simulink model "tx2"  (R2022a)
settings: Solver=FixedStepDiscrete  StartTime=0.0  StopTime=3.1e6  FixedStep=1  RelTol=1e-3
undefined symbols (not defined in the file or in its folder): rom_bf1, rom_bf2, rom_bf3, rom_bf4, rom_bf5, rom_bf6, rom_bf7, rom_bf8, rom_pilot_tt
libraries: hdlsllib x809, whdlutilities x460, whdlmod x104, whdledac x26, simulink x3
(part 9 of 27)

== system tx2/Subsystem9/bit_level ==
  note: 此时的输出本身具有一位延迟
  process_data : Inport
  process_valid : Inport  Port=2  OutDataTypeStr=Bus: samplecontrol
  Compare To Constant1 : hdlsllib/Logic and Bit Operations/Compare To Constant  relop=<  const=385  OutDataTypeStr=boolean
      settings: SourceProductBaseCode=SL
  Compare To Constant2 : hdlsllib/Logic and Bit Operations/Compare To Constant  relop===  const=1584+192  OutDataTypeStr=boolean
      settings: SourceProductBaseCode=SL
  Compare To Constant3 : hdlsllib/Logic and Bit Operations/Compare To Constant  relop=>  const=576  OutDataTypeStr=boolean
      settings: SourceProductBaseCode=SL
  Compare To Constant4 : hdlsllib/Logic and Bit Operations/Compare To Constant  relop=<=  const=1584+192  OutDataTypeStr=boolean
      settings: SourceProductBaseCode=SL
  Compare To Constant5 : hdlsllib/Logic and Bit Operations/Compare To Constant  relop=>=  const=792+1  OutDataTypeStr=boolean
      settings: SourceProductBaseCode=SL
  Compare To Constant6 : hdlsllib/Logic and Bit Operations/Compare To Constant  relop=<=  const=1584  OutDataTypeStr=boolean
      settings: SourceProductBaseCode=SL
  Constant : Constant  OutDataTypeStr=boolean
  Constant1 : Constant  Value=72  OutDataTypeStr=uint16
  Constant2 : Constant  Value=0  OutDataTypeStr=boolean
  Constant3 : Constant  Value=0  OutDataTypeStr=fixdt(0,12,0)
  Data Type Conversion1 : DataTypeConversion  OutDataTypeStr=fixdt(0,1,0)  SaturateOnIntegerOverflow=off  RndMeth=Floor
  Data Type Conversion2 : DataTypeConversion  OutDataTypeStr=boolean  SaturateOnIntegerOverflow=off  RndMeth=Floor
  Data Type Conversion3 : DataTypeConversion  OutDataTypeStr=boolean  SaturateOnIntegerOverflow=off  RndMeth=Floor
  Delay1 : Delay  DelayLength=1  InitialCondition=0
  Delay2 : Delay  DelayLength=1  InitialCondition=0
  HDL Counter1 : hdlsllib/Sources/HDL Counter  CountType=Count limited  CountInit=1  CountStep=1  CountMax=1584  CountFromType=Initial value  CountFrom=1  CountResetPort=on  CountLoadPort=off  CountEnbPort=on  CountDirPort=off  CountHitOutputPort=off  CountDataType=Unsigned  CountWordLen=12  CountFracLen=0  CountSampTime=1
  HDL Counter2 : hdlsllib/Sources/HDL Counter  CountType=Count limited  CountInit=1  CountStep=1  CountMax=792  CountFromType=Initial value  CountFrom=1  CountResetPort=on  CountLoadPort=off  CountEnbPort=on  CountDirPort=off  CountHitOutputPort=off  CountDataType=Unsigned  CountWordLen=12  CountFracLen=0  CountSampTime=1
  HDL Counter4 : hdlsllib/Sources/HDL Counter  CountType=Count limited  CountInit=1  CountStep=1  CountMax=4096-1  CountFromType=Initial value  CountFrom=1  CountResetPort=on  CountLoadPort=off  CountEnbPort=on  CountDirPort=off  CountHitOutputPort=off  CountDataType=Unsigned  CountWordLen=12  CountFracLen=0  CountSampTime=1
  HDL Counter5 : hdlsllib/Sources/HDL Counter  CountType=Count limited  CountInit=0  CountStep=1  CountMax=1  CountFromType=Initial value  CountFrom=0  CountResetPort=on  CountLoadPort=off  CountEnbPort=on  CountDirPort=off  CountHitOutputPort=off  CountDataType=Unsigned  CountWordLen=1  CountFracLen=0  CountSampTime=1
  Logical Operator : Logic  Operator=OR  AllPortsSameDT=off  OutDataTypeStr=boolean
  Logical Operator{1,3,7..8} (4 alike) : Logic  Operator=NOT  AllPortsSameDT=off  OutDataTypeStr=boolean
  Logical Operator{2,4..6} (4 alike) : Logic  AllPortsSameDT=off  OutDataTypeStr=boolean
  Mux : Mux  Inputs=2
  NR CRC Encoder : whdledac/NR CRC Encoder  CRCType=CRC16  EnableCRCMaskPort=off  SimulateUsing=Code generation
      settings: SourceProductBaseCode=LH
  NR LDPC Encoder2 : whdledac/NR LDPC Encoder
      settings: SourceProductBaseCode=LH
  Sample Control Bus Creator : whdlutilities/Sample Control Bus Creator
      settings: SourceProductBaseCode=LH
  Sample Control Bus Selector : whdlutilities/Sample Control Bus Selector  OutputSignals=start,end,valid
      settings: SourceProductBaseCode=LH
  Sample Control Bus Selector1 : whdlutilities/Sample Control Bus Selector  OutputSignals=start,end,valid
      settings: SourceProductBaseCode=LH
  Simple Dual Port RAM1 : hdlsllib/HDL RAMs/Simple Dual Port RAM  ram_size=12
      settings: SourceProductBaseCode=SL
  Subsystem : Subsystem
  Switch : Switch  Criteria=u2 ~= 0  SaturateOnIntegerOverflow=off  InputSameDT=off
  Switch1 : Switch  Criteria=u2 ~= 0  SaturateOnIntegerOverflow=off  InputSameDT=off
  Switch2 : Switch  Criteria=u2 ~= 0  SaturateOnIntegerOverflow=off  InputSameDT=off
  ctrl_gen : Subsystem
  valid_recover : Subsystem
  bit_level_process : Outport  OutDataTypeStr=boolean
  "bit_level_ctrl_process " : Outport  Port=2  OutDataTypeStr=Bus: samplecontrol
  wires:
  ctrl_gen/1(data_out) -> bit_level_process/1  "INTERLEAVE"
  process_valid/1 -> NR CRC Encoder/2
  Delay2/1 -> ctrl_gen/2(select_valid)
  Delay1/1 -> Mux/2
  Compare To Constant4/1 -> Logical Operator2/2
  Mux/1 -> ctrl_gen/1(data_in)
  Sample Control Bus Creator/1 -> NR LDPC Encoder2/2
  NR CRC Encoder/2 -> Sample Control Bus Selector/1
  Compare To Constant1/1 -> Logical Operator/1
  Compare To Constant2/1 -> HDL Counter5/2
  Constant2/1 -> Switch/3
  Compare To Constant6/1 -> Logical Operator6/2
  HDL Counter4/1 -> Compare To Constant2/1, Compare To Constant3/1, Compare To Constant4/1, Compare To Constant1/1  "wr_addr"
  Data Type Conversion1/1 -> Simple Dual Port RAM1/1  "wr_din"
  Compare To Constant5/1 -> Logical Operator6/1
  Logical Operator5/1 -> Simple Dual Port RAM1/3, Switch1/2, HDL Counter1/2  "wr_en"
  Compare To Constant3/1 -> Logical Operator/2
  Subsystem/1(end_out) -> valid_recover/3(end_in)
  process_data/1 -> NR CRC Encoder/1
  Data Type Conversion2/1 -> HDL Counter4/1
  Switch1/1 -> Simple Dual Port RAM1/2  "wr_addr"
  Logical Operator6/1 -> Switch/2, Delay2/1, Logical Operator7/1, Switch2/2, HDL Counter2/2
  Logical Operator1/1 -> HDL Counter1/1
  valid_recover/1(data_out) -> NR LDPC Encoder2/1
  NR LDPC Encoder2/2 -> Sample Control Bus Selector1/1
  HDL Counter1/1 -> Compare To Constant5/1, Compare To Constant6/1, Switch1/1
  Switch2/1 -> Simple Dual Port RAM1/4  "rd_addr"
  valid_recover/4(valid_out) -> Sample Control Bus Creator/3
  Logical Operator/1 -> Logical Operator2/1
  Logical Operator4/1 -> Logical Operator5/2
  Logical Operator3/1 -> Logical Operator4/1
  Logical Operator7/1 -> HDL Counter2/1
  Logical Operator2/1 -> Logical Operator5/1
  Sample Control Bus Selector1/3 -> Logical Operator4/2, Logical Operator1/1, Logical Operator8/1, HDL Counter4/2  "<valid>"
  valid_recover/3(end_out) -> Sample Control Bus Creator/2
  valid_recover/2(start_out) -> Sample Control Bus Creator/1
  Sample Control Bus Selector/1 -> valid_recover/2(start_in)  "<start>"
  Simple Dual Port RAM1/1 -> Data Type Conversion3/1
  NR LDPC Encoder2/1 -> Data Type Conversion1/1, Switch/1  "LDPC"
  Sample Control Bus Selector/2 -> Subsystem/1(end_in)  "<end>"
  Logical Operator8/1 -> HDL Counter5/1
  HDL Counter2/1 -> Switch2/1  "rd_addr"
  Constant1/1 -> NR LDPC Encoder2/4
  ctrl_gen/2(ctrl_out) -> "bit_level_ctrl_process "/1
  NR CRC Encoder/1 -> valid_recover/1(data_in)  "CRC"
  Constant3/1 -> Switch1/3, Switch2/3
  Constant/1 -> NR LDPC Encoder2/3
  Data Type Conversion3/1 -> Mux/1
  HDL Counter5/1 -> Data Type Conversion2/1, Logical Operator3/1  "loop_ctrl"
  Switch/1 -> Delay1/1

== system tx2/Subsystem9/mapping_process_L1 ==
  data_in : Inport  OutDataTypeStr=boolean
  mapping_ctrl : Inport  Port=2  OutDataTypeStr=Bus: samplecontrol
  Constant : Constant  Value=sqrt(2)/2  OutDataTypeStr=fixdt(1,16,14)
  Constant1 : Constant  Value=-sqrt(2)/2  OutDataTypeStr=fixdt(1,16,14)
  Constant2 : Constant  Value=0  OutDataTypeStr=uint8
  Constant3 : Constant  Value=0  OutDataTypeStr=fixdt(1,16,14)
  Delay : Delay  DelayLength=1  InitialCondition=0  ShowEnablePort=on
      settings: InputPortMap=u0,e6
  Delay{1,5..8,10..12} (8 alike) : Delay  DelayLength=1  InitialCondition=0
  Delay{3..4,9,13} (4 alike) : Delay  InitialCondition=0
  Delay2 : Delay  DelayLength=1  InitialCondition=0  ShowEnablePort=on
      settings: InputPortMap=u0,e6
  Demux : Demux  Outputs=2
  Logical Operator : Logic  Operator=OR  AllPortsSameDT=off  OutDataTypeStr=boolean
  Logical Operator1 : Logic  AllPortsSameDT=off  OutDataTypeStr=boolean
  Logical Operator13 : Logic  Operator=NOT  AllPortsSameDT=off  OutDataTypeStr=boolean
  Real-Imag to Complex : RealImagToComplex
  Real-Imag to Complex1 : RealImagToComplex
  Sample Control Bus Creator : whdlutilities/Sample Control Bus Creator
      settings: SourceProductBaseCode=LH
  Sample Control Bus Creator1 : whdlutilities/Sample Control Bus Creator
      settings: SourceProductBaseCode=LH
  Sample Control Bus Selector : whdlutilities/Sample Control Bus Selector  OutputSignals=start,end,valid
      settings: SourceProductBaseCode=LH
  Switch{,1..3} (4 alike) : Switch  Criteria=u2 ~= 0  SaturateOnIntegerOverflow=off  InputSameDT=off
  "divide6 " : hdlsllib/Sources/HDL Counter  CountType=Count limited  CountInit=1  CountStep=1  CountMax=12  CountFromType=Initial value  CountFrom=1  CountResetPort=on  CountLoadPort=off  CountEnbPort=on  CountDirPort=off  CountHitOutputPort=on  CountDataType=Unsigned  CountWordLen=8  CountFracLen=0  CountSampTime=1
  divide6 1 : hdlsllib/Sources/HDL Counter  CountType=Count limited  CountInit=1  CountStep=1  CountMax=6*12  CountFromType=Initial value  CountFrom=1  CountResetPort=on  CountLoadPort=off  CountEnbPort=on  CountDirPort=off  CountHitOutputPort=off  CountDataType=Unsigned  CountWordLen=8  CountFracLen=0  CountSampTime=1
  data_out : Outport  VectorParamsAs1DForOutWhenUnconnected=off
      settings: SignalType=complex
  ctrl_mapping : Outport  Port=2  OutDataTypeStr=Bus: samplecontrol  VectorParamsAs1DForOutWhenUnconnected=off
  RB_ctrl : Outport  Port=3  OutDataTypeStr=Bus: samplecontrol  VectorParamsAs1DForOutWhenUnconnected=off
  RB_id : Outport  Port=4  OutDataTypeStr=uint8  VectorParamsAs1DForOutWhenUnconnected=off
  wires:
  Constant1/1 -> Switch1/1, Switch/1
  Constant/1 -> Switch/3, Switch1/3
  Delay13/1 -> Switch3/2
  Real-Imag to Complex1/1 -> Switch3/3
  Constant3/1 -> Real-Imag to Complex1/1, Real-Imag to Complex1/2
  Switch3/1 -> data_out/1
  data_in/1 -> Delay/1  "data_with_CP"
  Sample Control Bus Creator1/1 -> RB_ctrl/1
  Delay7/1 -> RB_id/1
  Delay5/1 -> ctrl_mapping/1
  Delay12/1 -> Sample Control Bus Creator1/3
  Delay11/1 -> Sample Control Bus Creator1/2
  Delay8/1 -> Sample Control Bus Creator1/1
  Logical Operator1/1 -> Delay8/1
  Delay10/1 -> Logical Operator/1
  Delay9/1 -> Logical Operator/2
  Logical Operator/1 -> Logical Operator1/2
  Delay6/1 -> Switch3/1
  Constant2/1 -> Switch2/3
  Switch2/1 -> Delay7/1
  Delay4/1 -> Logical Operator1/1, Switch2/2, Delay12/1, "divide6 "/2, Logical Operator13/1
  divide6 1/1 -> Switch2/1  "RB_id"
  Sample Control Bus Creator/1 -> Delay3/1
  Sample Control Bus Selector/3 -> Delay/2, Delay1/1, Delay4/1, Sample Control Bus Creator/3  "<valid>"
  Sample Control Bus Selector/2 -> Sample Control Bus Creator/2  "<end>"
  Sample Control Bus Selector/1 -> Sample Control Bus Creator/1, Delay9/1  "<start>"
  Logical Operator13/1 -> "divide6 "/1, divide6 1/1
  "divide6 "/2 -> Delay10/1, Delay11/1, divide6 1/2  "count6"
  mapping_ctrl/1 -> Sample Control Bus Selector/1
  Delay1/1 -> Delay13/1, Delay2/2
  Delay3/1 -> Delay5/1
  Delay2/1 -> Delay6/1
  Real-Imag to Complex/1 -> Delay2/1
  Demux/2 -> Switch1/2
  Demux/1 -> Switch/2
  Delay/1 -> Demux/1
  Switch/1 -> Real-Imag to Complex/1
  Switch1/1 -> Real-Imag to Complex/2

== system tx2/transport_block1/Subsystem10 ==
  data_in : Inport
  select_valid : Inport  Port=2  OutDataTypeStr=boolean
  Constant : Constant  Value=0  OutDataTypeStr=boolean
  Switch : Switch  Criteria=u2 ~= 0  SaturateOnIntegerOverflow=off  InputSameDT=off
  ctrl_gen : Subsystem
  data_out : Outport
  ctrl_out : Outport  Port=2
  wires:
  Switch/1 -> ctrl_gen/1(data_in)
  Constant/1 -> Switch/3
  select_valid/1 -> ctrl_gen/2(valid_in), Switch/2
  ctrl_gen/1(data_out) -> data_out/1
  ctrl_gen/2(ctrl_out) -> ctrl_out/1
  data_in/1 -> Switch/1

== system tx2/transport_block1/Subsystem11 ==
  data_in : Inport
  select_valid : Inport  Port=2  OutDataTypeStr=boolean
  Constant : Constant  Value=0  OutDataTypeStr=boolean
  Switch : Switch  Criteria=u2 ~= 0  SaturateOnIntegerOverflow=off  InputSameDT=off
  ctrl_gen : Subsystem
  data_out : Outport
  ctrl_out : Outport  Port=2
  wires:
  data_in/1 -> Switch/1
  ctrl_gen/2(ctrl_out) -> ctrl_out/1
  ctrl_gen/1(data_out) -> data_out/1
  select_valid/1 -> Switch/2, ctrl_gen/2(valid_in)
  Constant/1 -> Switch/3
  Switch/1 -> ctrl_gen/1(data_in)

== system tx2/transport_block1/Subsystem12 ==
  data_in : Inport
  select_valid : Inport  Port=2  OutDataTypeStr=boolean
  Constant : Constant  Value=0  OutDataTypeStr=boolean
  Switch : Switch  Criteria=u2 ~= 0  SaturateOnIntegerOverflow=off  InputSameDT=off
  ctrl_gen : Subsystem
  data_out : Outport
  ctrl_out : Outport  Port=2
  wires:
  Switch/1 -> ctrl_gen/1(data_in)
  Constant/1 -> Switch/3
  select_valid/1 -> ctrl_gen/2(valid_in), Switch/2
  ctrl_gen/1(data_out) -> data_out/1
  ctrl_gen/2(ctrl_out) -> ctrl_out/1
  data_in/1 -> Switch/1

== system tx2/transport_block1/Subsystem13 ==
  data_in : Inport
  select_valid : Inport  Port=2  OutDataTypeStr=boolean
  Constant : Constant  Value=0  OutDataTypeStr=boolean
  Switch : Switch  Criteria=u2 ~= 0  SaturateOnIntegerOverflow=off  InputSameDT=off
  ctrl_gen : Subsystem
  data_out : Outport
  ctrl_out : Outport  Port=2
  wires:
  data_in/1 -> Switch/1
  ctrl_gen/2(ctrl_out) -> ctrl_out/1
  ctrl_gen/1(data_out) -> data_out/1
  select_valid/1 -> Switch/2, ctrl_gen/2(valid_in)
  Constant/1 -> Switch/3
  Switch/1 -> ctrl_gen/1(data_in)

== system tx2/transport_block1/Subsystem14 ==
  data_in : Inport
  select_valid : Inport  Port=2  OutDataTypeStr=boolean
  Constant : Constant  Value=0  OutDataTypeStr=boolean
  Switch : Switch  Criteria=u2 ~= 0  SaturateOnIntegerOverflow=off  InputSameDT=off
  ctrl_gen : Subsystem
  data_out : Outport
  ctrl_out : Outport  Port=2
  wires:
  Switch/1 -> ctrl_gen/1(data_in)
  Constant/1 -> Switch/3
  select_valid/1 -> ctrl_gen/2(valid_in), Switch/2
  ctrl_gen/1(data_out) -> data_out/1
  ctrl_gen/2(ctrl_out) -> ctrl_out/1
  data_in/1 -> Switch/1

== system tx2/transport_block1/Subsystem2 ==
  data_in : Inport
  select_valid : Inport  Port=2  OutDataTypeStr=boolean
  Constant : Constant  Value=0  OutDataTypeStr=boolean
  Switch : Switch  Criteria=u2 ~= 0  SaturateOnIntegerOverflow=off  InputSameDT=off
  ctrl_gen : Subsystem
  data_out : Outport
  ctrl_out : Outport  Port=2
  wires:
  data_in/1 -> Switch/1
  ctrl_gen/2(ctrl_out) -> ctrl_out/1
  ctrl_gen/1(data_out) -> data_out/1
  select_valid/1 -> Switch/2, ctrl_gen/2(valid_in)
  Constant/1 -> Switch/3
  Switch/1 -> ctrl_gen/1(data_in)

== system tx2/transport_block1/Subsystem3 ==
  data_in : Inport
  select_valid : Inport  Port=2  OutDataTypeStr=boolean
  Constant : Constant  Value=0  OutDataTypeStr=boolean
  Switch : Switch  Criteria=u2 ~= 0  SaturateOnIntegerOverflow=off  InputSameDT=off
  ctrl_gen : Subsystem
  data_out : Outport
  ctrl_out : Outport  Port=2
  wires:
  Switch/1 -> ctrl_gen/1(data_in)
  Constant/1 -> Switch/3
  select_valid/1 -> ctrl_gen/2(valid_in), Switch/2
  ctrl_gen/1(data_out) -> data_out/1
  ctrl_gen/2(ctrl_out) -> ctrl_out/1
  data_in/1 -> Switch/1

== system tx2/transport_block1/Subsystem4 ==
  data_in : Inport
  select_valid : Inport  Port=2  OutDataTypeStr=boolean
  Constant : Constant  Value=0  OutDataTypeStr=boolean
  Switch : Switch  Criteria=u2 ~= 0  SaturateOnIntegerOverflow=off  InputSameDT=off
  ctrl_gen : Subsystem
  data_out : Outport
  ctrl_out : Outport  Port=2
  wires:
  data_in/1 -> Switch/1
  ctrl_gen/2(ctrl_out) -> ctrl_out/1
  ctrl_gen/1(data_out) -> data_out/1
  select_valid/1 -> Switch/2, ctrl_gen/2(valid_in)
  Constant/1 -> Switch/3
  Switch/1 -> ctrl_gen/1(data_in)

== system tx2/transport_block1/Subsystem5 ==
  data_in : Inport
  select_valid : Inport  Port=2  OutDataTypeStr=boolean
  Constant : Constant  Value=0  OutDataTypeStr=boolean
  Switch : Switch  Criteria=u2 ~= 0  SaturateOnIntegerOverflow=off  InputSameDT=off
  ctrl_gen : Subsystem
  data_out : Outport
  ctrl_out : Outport  Port=2
  wires:
  Switch/1 -> ctrl_gen/1(data_in)
  Constant/1 -> Switch/3
  select_valid/1 -> ctrl_gen/2(valid_in), Switch/2
  ctrl_gen/1(data_out) -> data_out/1
  ctrl_gen/2(ctrl_out) -> ctrl_out/1
  data_in/1 -> Switch/1

== system tx2/transport_block1/Subsystem6 ==
  data_in : Inport
  select_valid : Inport  Port=2  OutDataTypeStr=boolean
  Constant : Constant  Value=0  OutDataTypeStr=boolean
  Switch : Switch  Criteria=u2 ~= 0  SaturateOnIntegerOverflow=off  InputSameDT=off
  ctrl_gen : Subsystem
  data_out : Outport
  ctrl_out : Outport  Port=2
  wires:
  data_in/1 -> Switch/1
  ctrl_gen/2(ctrl_out) -> ctrl_out/1
  ctrl_gen/1(data_out) -> data_out/1
  select_valid/1 -> Switch/2, ctrl_gen/2(valid_in)
  Constant/1 -> Switch/3
  Switch/1 -> ctrl_gen/1(data_in)

== system tx2/transport_block1/Subsystem7 ==
  data_in : Inport
  select_valid : Inport  Port=2  OutDataTypeStr=boolean
  Constant : Constant  Value=0  OutDataTypeStr=boolean
  Switch : Switch  Criteria=u2 ~= 0  SaturateOnIntegerOverflow=off  InputSameDT=off
  ctrl_gen : Subsystem
  data_out : Outport
  ctrl_out : Outport  Port=2
  wires:
  Switch/1 -> ctrl_gen/1(data_in)
  Constant/1 -> Switch/3
  select_valid/1 -> ctrl_gen/2(valid_in), Switch/2
  ctrl_gen/1(data_out) -> data_out/1
  ctrl_gen/2(ctrl_out) -> ctrl_out/1
  data_in/1 -> Switch/1

== system tx2/transport_block1/Subsystem8 ==
  data_in : Inport
  select_valid : Inport  Port=2  OutDataTypeStr=boolean
  Constant : Constant  Value=0  OutDataTypeStr=boolean
  Switch : Switch  Criteria=u2 ~= 0  SaturateOnIntegerOverflow=off  InputSameDT=off
  ctrl_gen : Subsystem
  data_out : Outport
  ctrl_out : Outport  Port=2
  wires:
  data_in/1 -> Switch/1
  ctrl_gen/2(ctrl_out) -> ctrl_out/1
  ctrl_gen/1(data_out) -> data_out/1
  select_valid/1 -> Switch/2, ctrl_gen/2(valid_in)
  Constant/1 -> Switch/3
  Switch/1 -> ctrl_gen/1(data_in)

== system tx2/transport_block1/Subsystem9 ==
  data_in : Inport
  select_valid : Inport  Port=2  OutDataTypeStr=boolean
  Constant : Constant  Value=0  OutDataTypeStr=boolean
  Switch : Switch  Criteria=u2 ~= 0  SaturateOnIntegerOverflow=off  InputSameDT=off
  ctrl_gen : Subsystem
  data_out : Outport
  ctrl_out : Outport  Port=2
  wires:
  data_in/1 -> Switch/1
  ctrl_gen/2(ctrl_out) -> ctrl_out/1
  ctrl_gen/1(data_out) -> data_out/1
  select_valid/1 -> Switch/2, ctrl_gen/2(valid_in)
  Constant/1 -> Switch/3
  Switch/1 -> ctrl_gen/1(data_in)

== system tx2/transport_block1/process_selector ==
  enb : Inport
  rst : Inport  Port=2  OutDataTypeStr=boolean
  Constant : Constant  Value=0  OutDataTypeStr=uint8
  HDL Counter : hdlsllib/Sources/HDL Counter  CountType=Count limited  CountInit=1  CountStep=1  CountMax=transblock_len  CountFromType=Initial value  CountFrom=1  CountResetPort=on  CountLoadPort=off  CountEnbPort=on  CountDirPort=off  CountHitOutputPort=on  CountDataType=Unsigned  CountWordLen=10  CountFracLen=0  CountSampTime=1
  HDL Counter1 : hdlsllib/Sources/HDL Counter  CountType=Count limited  CountInit=1  CountStep=1  CountMax=process_len  CountFromType=Initial value  CountFrom=1  CountResetPort=on  CountLoadPort=off  CountEnbPort=on  CountDirPort=off  CountHitOutputPort=off  CountDataType=Unsigned  CountWordLen=8  CountFracLen=0  CountSampTime=1
  Switch : Switch  Criteria=u2 ~= 0  SaturateOnIntegerOverflow=off  InputSameDT=off
  selector : Outport
  wires:
  rst/1 -> HDL Counter1/1, HDL Counter/1
  HDL Counter1/1 -> Switch/1
  enb/1 -> HDL Counter/2, Switch/2
  HDL Counter/1 -> ?
  Switch/1 -> selector/1
  Constant/1 -> Switch/3
  HDL Counter/2 -> HDL Counter1/2

== system tx2/Subsystem1/BF/rom_bf1 ==
  address : Inport
  read_en : Inport  Port=2
  HDL ROM : Subsystem
  InputReg : Delay  DelayLength=1  ShowEnablePort=on
      settings: InputPortMap=u0,e6
  data_out : Outport
  wires:
  address/1 -> InputReg/1
  InputReg/1 -> HDL ROM/1(rom_address)
  read_en/1 -> InputReg/2
  HDL ROM/1(data_out) -> data_out/1

== system tx2/Subsystem1/BF/rom_bf2 ==
  address : Inport
  read_en : Inport  Port=2
  HDL ROM : Subsystem
  InputReg : Delay  DelayLength=1  ShowEnablePort=on
      settings: InputPortMap=u0,e6
  data_out : Outport
  wires:
  HDL ROM/1(data_out) -> data_out/1
  read_en/1 -> InputReg/2
  InputReg/1 -> HDL ROM/1(rom_address)
  address/1 -> InputReg/1

== system tx2/Subsystem1/BF/rom_bf3 ==
  address : Inport
  read_en : Inport  Port=2
  HDL ROM : Subsystem
  InputReg : Delay  DelayLength=1  ShowEnablePort=on
      settings: InputPortMap=u0,e6
  data_out : Outport
  wires:
  address/1 -> InputReg/1
  InputReg/1 -> HDL ROM/1(rom_address)
  read_en/1 -> InputReg/2
  HDL ROM/1(data_out) -> data_out/1

== system tx2/Subsystem1/BF/rom_bf4 ==
  address : Inport
  read_en : Inport  Port=2
  HDL ROM : Subsystem
  InputReg : Delay  DelayLength=1  ShowEnablePort=on
      settings: InputPortMap=u0,e6
  data_out : Outport
  wires:
  HDL ROM/1(data_out) -> data_out/1
  read_en/1 -> InputReg/2
  InputReg/1 -> HDL ROM/1(rom_address)
  address/1 -> InputReg/1

== system tx2/Subsystem1/BF/rom_bf5 ==
  address : Inport
  read_en : Inport  Port=2
  HDL ROM : Subsystem
  InputReg : Delay  DelayLength=1  ShowEnablePort=on
      settings: InputPortMap=u0,e6
  data_out : Outport
  wires:
  address/1 -> InputReg/1
  InputReg/1 -> HDL ROM/1(rom_address)
  read_en/1 -> InputReg/2
  HDL ROM/1(data_out) -> data_out/1

== system tx2/Subsystem1/BF/rom_bf6 ==
  address : Inport
  read_en : Inport  Port=2
  HDL ROM : Subsystem
  InputReg : Delay  DelayLength=1  ShowEnablePort=on
      settings: InputPortMap=u0,e6
  data_out : Outport
  wires:
  HDL ROM/1(data_out) -> data_out/1
  read_en/1 -> InputReg/2
  InputReg/1 -> HDL ROM/1(rom_address)
  address/1 -> InputReg/1

== system tx2/Subsystem1/BF/rom_bf7 ==
  address : Inport
  read_en : Inport  Port=2
  HDL ROM : Subsystem
  InputReg : Delay  DelayLength=1  ShowEnablePort=on
      settings: InputPortMap=u0,e6
  data_out : Outport
  wires:
  address/1 -> InputReg/1
  InputReg/1 -> HDL ROM/1(rom_address)
  read_en/1 -> InputReg/2
  HDL ROM/1(data_out) -> data_out/1

== system tx2/Subsystem1/BF/rom_bf8 ==
  address : Inport
  read_en : Inport  Port=2
  HDL ROM : Subsystem
  InputReg : Delay  DelayLength=1  ShowEnablePort=on
      settings: InputPortMap=u0,e6
  data_out : Outport
  wires:
  HDL ROM/1(data_out) -> data_out/1
  read_en/1 -> InputReg/2
  InputReg/1 -> HDL ROM/1(rom_address)
  address/1 -> InputReg/1

== system tx2/Subsystem1/OFDM_process1/OFDM_process1_bf1 ==
  data : Inport
  BF_ctrl : Inport  Port=2
  OFDM_BF1 : Subsystem
  ctrl_gen : Subsystem
  OFDM_process : Outport
  OFDM_ctrl_process : Outport  Port=2
  wires:
  OFDM_BF1/1(data_out) -> ctrl_gen/1(data_in)
  OFDM_BF1/2(valid_out) -> ctrl_gen/2(valid_in)
  data/1 -> OFDM_BF1/1(data)
  ctrl_gen/2(ctrl_out) -> OFDM_ctrl_process/1  "OFDM_ctrl_bf1_process1"
  BF_ctrl/1 -> OFDM_BF1/2(OFDM_ctrl)
  ctrl_gen/1(data_out) -> OFDM_process/1  "OFDM_bf1_process1"

== system tx2/Subsystem1/OFDM_process1/OFDM_process1_bf2 ==
  data : Inport
  BF_ctrl : Inport  Port=2
  OFDM_BF1 : Subsystem
  ctrl_gen : Subsystem
  OFDM_process : Outport
  OFDM_ctrl_process : Outport  Port=2
  wires:
  ctrl_gen/1(data_out) -> OFDM_process/1  "OFDM_bf1_process1"
  BF_ctrl/1 -> OFDM_BF1/2(OFDM_ctrl)
  ctrl_gen/2(ctrl_out) -> OFDM_ctrl_process/1  "OFDM_ctrl_bf1_process1"
  data/1 -> OFDM_BF1/1(data)
  OFDM_BF1/2(valid_out) -> ctrl_gen/2(valid_in)
  OFDM_BF1/1(data_out) -> ctrl_gen/1(data_in)

== system tx2/Subsystem1/OFDM_process1/OFDM_process1_bf3 ==
  data : Inport
  BF_ctrl : Inport  Port=2
  OFDM_BF1 : Subsystem
  ctrl_gen : Subsystem
  OFDM_process : Outport
  OFDM_ctrl_process : Outport  Port=2
  wires:
  OFDM_BF1/1(data_out) -> ctrl_gen/1(data_in)
  OFDM_BF1/2(valid_out) -> ctrl_gen/2(valid_in)
  data/1 -> OFDM_BF1/1(data)
  ctrl_gen/2(ctrl_out) -> OFDM_ctrl_process/1  "OFDM_ctrl_bf1_process1"
  BF_ctrl/1 -> OFDM_BF1/2(OFDM_ctrl)
  ctrl_gen/1(data_out) -> OFDM_process/1  "OFDM_bf1_process1"

== system tx2/Subsystem1/OFDM_process1/OFDM_process1_bf4 ==
  data : Inport
  BF_ctrl : Inport  Port=2
  OFDM_BF1 : Subsystem
  ctrl_gen : Subsystem
  OFDM_process : Outport
  OFDM_ctrl_process : Outport  Port=2
  wires:
  ctrl_gen/1(data_out) -> OFDM_process/1  "OFDM_bf1_process1"
  BF_ctrl/1 -> OFDM_BF1/2(OFDM_ctrl)
  ctrl_gen/2(ctrl_out) -> OFDM_ctrl_process/1  "OFDM_ctrl_bf1_process1"
  data/1 -> OFDM_BF1/1(data)
  OFDM_BF1/2(valid_out) -> ctrl_gen/2(valid_in)
  OFDM_BF1/1(data_out) -> ctrl_gen/1(data_in)

== system tx2/Subsystem1/OFDM_process1/OFDM_process1_bf5 ==
  data : Inport
  BF_ctrl : Inport  Port=2
  OFDM_BF1 : Subsystem
  ctrl_gen : Subsystem
  OFDM_process : Outport
  OFDM_ctrl_process : Outport  Port=2
  wires:
  OFDM_BF1/1(data_out) -> ctrl_gen/1(data_in)
  OFDM_BF1/2(valid_out) -> ctrl_gen/2(valid_in)
  data/1 -> OFDM_BF1/1(data)
  ctrl_gen/2(ctrl_out) -> OFDM_ctrl_process/1  "OFDM_ctrl_bf1_process1"
  BF_ctrl/1 -> OFDM_BF1/2(OFDM_ctrl)
  ctrl_gen/1(data_out) -> OFDM_process/1  "OFDM_bf1_process1"

== system tx2/Subsystem1/OFDM_process1/OFDM_process1_bf6 ==
  data : Inport
  BF_ctrl : Inport  Port=2
  OFDM_BF1 : Subsystem
  ctrl_gen : Subsystem
  OFDM_process : Outport
  OFDM_ctrl_process : Outport  Port=2
  wires:
  ctrl_gen/1(data_out) -> OFDM_process/1  "OFDM_bf1_process1"
  BF_ctrl/1 -> OFDM_BF1/2(OFDM_ctrl)
  ctrl_gen/2(ctrl_out) -> OFDM_ctrl_process/1  "OFDM_ctrl_bf1_process1"
  data/1 -> OFDM_BF1/1(data)
  OFDM_BF1/2(valid_out) -> ctrl_gen/2(valid_in)
  OFDM_BF1/1(data_out) -> ctrl_gen/1(data_in)

== system tx2/Subsystem1/OFDM_process1/OFDM_process1_bf7 ==
  data : Inport
  BF_ctrl : Inport  Port=2
  OFDM_BF1 : Subsystem
  ctrl_gen : Subsystem
  OFDM_process : Outport
  OFDM_ctrl_process : Outport  Port=2
  wires:
  OFDM_BF1/1(data_out) -> ctrl_gen/1(data_in)
  OFDM_BF1/2(valid_out) -> ctrl_gen/2(valid_in)
  data/1 -> OFDM_BF1/1(data)
  ctrl_gen/2(ctrl_out) -> OFDM_ctrl_process/1  "OFDM_ctrl_bf1_process1"
  BF_ctrl/1 -> OFDM_BF1/2(OFDM_ctrl)
  ctrl_gen/1(data_out) -> OFDM_process/1  "OFDM_bf1_process1"

== system tx2/Subsystem1/OFDM_process1/OFDM_process1_bf8 ==
  data : Inport
  BF_ctrl : Inport  Port=2
  OFDM_BF1 : Subsystem
  ctrl_gen : Subsystem
  OFDM_process : Outport
  OFDM_ctrl_process : Outport  Port=2
  wires:
  ctrl_gen/1(data_out) -> OFDM_process/1  "OFDM_bf1_process1"
  BF_ctrl/1 -> OFDM_BF1/2(OFDM_ctrl)
  ctrl_gen/2(ctrl_out) -> OFDM_ctrl_process/1  "OFDM_ctrl_bf1_process1"
  data/1 -> OFDM_BF1/1(data)
  OFDM_BF1/2(valid_out) -> ctrl_gen/2(valid_in)
  OFDM_BF1/1(data_out) -> ctrl_gen/1(data_in)

== system tx2/Subsystem1/bit_level/Subsystem ==
  end_in : Inport  OutDataTypeStr=boolean
  Data Type Conversion : DataTypeConversion  OutDataTypeStr=boolean  SaturateOnIntegerOverflow=off  RndMeth=Floor
  HDL Counter : hdlsllib/Sources/HDL Counter  CountType=Count limited  CountInit=1  CountStep=1  CountMax=192  CountFromType=Initial value  CountFrom=1  CountResetPort=on  CountLoadPort=off  CountEnbPort=off  CountDirPort=off  CountHitOutputPort=on  CountDataType=Unsigned  CountWordLen=8  CountFracLen=0  CountSampTime=1
  HDL Counter1 : hdlsllib/Sources/HDL Counter  CountType=Count limited  CountInit=0  CountStep=1  CountMax=1  CountFromType=Initial value  CountFrom=0  CountResetPort=on  CountLoadPort=off  CountEnbPort=on  CountDirPort=off  CountHitOutputPort=off  CountDataType=Unsigned  CountWordLen=1  CountFracLen=0  CountSampTime=1
  Logical Operator : Logic  AllPortsSameDT=off  OutDataTypeStr=boolean
  end_out : Outport  OutDataTypeStr=boolean
  wires:
  HDL Counter1/1 -> Data Type Conversion/1
  end_in/1 -> HDL Counter/1, HDL Counter1/2
  Data Type Conversion/1 -> Logical Operator/2
  HDL Counter/2 -> Logical Operator/1, HDL Counter1/1
  Logical Operator/1 -> end_out/1

== system tx2/Subsystem1/bit_level/ctrl_gen ==
  data_in : Inport
  select_valid : Inport  Port=2  OutDataTypeStr=boolean
  Constant : Constant  Value=0  OutDataTypeStr=boolean
  Switch : Switch  Criteria=u2 ~= 0  SaturateOnIntegerOverflow=off  InputSameDT=off
  ctrl_gen : Subsystem
  data_out : Outport
  ctrl_out : Outport  Port=2
  wires:
  Switch/1 -> ctrl_gen/1(data_in)
  Constant/1 -> Switch/3
  select_valid/1 -> ctrl_gen/2(valid_in), Switch/2
  ctrl_gen/1(data_out) -> data_out/1
  ctrl_gen/2(ctrl_out) -> ctrl_out/1
  data_in/1 -> Switch/1

== system tx2/Subsystem1/bit_level/valid_recover ==
  data_in : Inport
  start_in : Inport  Port=2
  end_in : Inport  Port=3
  Constant : Constant  OutDataTypeStr=boolean
  Constant1 : Constant  Value=0  OutDataTypeStr=boolean
  Constant2 : Constant  OutDataTypeStr=boolean
  Constant3 : Constant  Value=0  OutDataTypeStr=boolean
  Constant4 : Constant  OutDataTypeStr=boolean
  Constant5 : Constant  Value=0  OutDataTypeStr=boolean
  Delay{,1..4} (5 alike) : Delay  DelayLength=1  InitialCondition=0
  Logical Operator1 : Logic  Operator=OR  AllPortsSameDT=off  OutDataTypeStr=boolean
  Logical Operator2 : Logic  AllPortsSameDT=off  OutDataTypeStr=boolean
  Switch : Switch  Criteria=u2 ~= 0  SaturateOnIntegerOverflow=off  InputSameDT=off
  Switch1 : Switch  Criteria=u2 ~= 0  SaturateOnIntegerOverflow=off  InputSameDT=off
  Switch2 : Switch  Criteria=u2 ~= 0  SaturateOnIntegerOverflow=off  InputSameDT=off
  data_out : Outport  VectorParamsAs1DForOutWhenUnconnected=off
  start_out : Outport  Port=2  VectorParamsAs1DForOutWhenUnconnected=off
  end_out : Outport  Port=3  VectorParamsAs1DForOutWhenUnconnected=off
  valid_out : Outport  Port=4  VectorParamsAs1DForOutWhenUnconnected=off
  wires:
  Delay4/1 -> data_out/1
  data_in/1 -> Delay4/1
  Delay1/1 -> Delay2/1, end_out/1
  end_in/1 -> Delay1/1
  Constant1/1 -> Switch/3
  Logical Operator2/1 -> Delay3/1, valid_out/1
  Constant3/1 -> Switch1/1
  start_in/1 -> Delay/1
  Constant4/1 -> Switch2/1
  Constant5/1 -> Switch2/3
  Delay3/1 -> Switch2/2
  Switch2/1 -> Logical Operator1/1
  Logical Operator1/1 -> Logical Operator2/1
  Delay2/1 -> Switch1/2
  Delay/1 -> Switch/2, start_out/1
  Switch1/1 -> Logical Operator2/2
  Switch/1 -> Logical Operator1/2
  Constant2/1 -> Switch1/3
  Constant/1 -> Switch/1

== system tx2/Subsystem10/BF/rom_bf1 ==
  address : Inport
  read_en : Inport  Port=2
  HDL ROM : Subsystem
  InputReg : Delay  DelayLength=1  ShowEnablePort=on
      settings: InputPortMap=u0,e6
  data_out : Outport
  wires:
  address/1 -> InputReg/1
  InputReg/1 -> HDL ROM/1(rom_address)
  read_en/1 -> InputReg/2
  HDL ROM/1(data_out) -> data_out/1

== system tx2/Subsystem10/BF/rom_bf2 ==
  address : Inport
  read_en : Inport  Port=2
  HDL ROM : Subsystem
  InputReg : Delay  DelayLength=1  ShowEnablePort=on
      settings: InputPortMap=u0,e6
  data_out : Outport
  wires:
  HDL ROM/1(data_out) -> data_out/1
  read_en/1 -> InputReg/2
  InputReg/1 -> HDL ROM/1(rom_address)
  address/1 -> InputReg/1

== system tx2/Subsystem10/BF/rom_bf3 ==
  address : Inport
  read_en : Inport  Port=2
  HDL ROM : Subsystem
  InputReg : Delay  DelayLength=1  ShowEnablePort=on
      settings: InputPortMap=u0,e6
  data_out : Outport
  wires:
  address/1 -> InputReg/1
  InputReg/1 -> HDL ROM/1(rom_address)
  read_en/1 -> InputReg/2
  HDL ROM/1(data_out) -> data_out/1

== system tx2/Subsystem10/BF/rom_bf4 ==
  address : Inport
  read_en : Inport  Port=2
  HDL ROM : Subsystem
  InputReg : Delay  DelayLength=1  ShowEnablePort=on
      settings: InputPortMap=u0,e6
  data_out : Outport
  wires:
  HDL ROM/1(data_out) -> data_out/1
  read_en/1 -> InputReg/2
  InputReg/1 -> HDL ROM/1(rom_address)
  address/1 -> InputReg/1

== system tx2/Subsystem10/BF/rom_bf5 ==
  address : Inport
  read_en : Inport  Port=2
  HDL ROM : Subsystem
  InputReg : Delay  DelayLength=1  ShowEnablePort=on
      settings: InputPortMap=u0,e6
  data_out : Outport
  wires:
  address/1 -> InputReg/1
  InputReg/1 -> HDL ROM/1(rom_address)
  read_en/1 -> InputReg/2
  HDL ROM/1(data_out) -> data_out/1

== system tx2/Subsystem10/BF/rom_bf6 ==
  address : Inport
  read_en : Inport  Port=2
  HDL ROM : Subsystem
  InputReg : Delay  DelayLength=1  ShowEnablePort=on
      settings: InputPortMap=u0,e6
  data_out : Outport
  wires:
  HDL ROM/1(data_out) -> data_out/1
  read_en/1 -> InputReg/2
  InputReg/1 -> HDL ROM/1(rom_address)
  address/1 -> InputReg/1

== system tx2/Subsystem10/BF/rom_bf7 ==
  address : Inport
  read_en : Inport  Port=2
  HDL ROM : Subsystem
  InputReg : Delay  DelayLength=1  ShowEnablePort=on
      settings: InputPortMap=u0,e6
  data_out : Outport
  wires:
  address/1 -> InputReg/1
  InputReg/1 -> HDL ROM/1(rom_address)
  read_en/1 -> InputReg/2
  HDL ROM/1(data_out) -> data_out/1

== system tx2/Subsystem10/BF/rom_bf8 ==
  address : Inport
  read_en : Inport  Port=2
  HDL ROM : Subsystem
  InputReg : Delay  DelayLength=1  ShowEnablePort=on
      settings: InputPortMap=u0,e6
  data_out : Outport
  wires:
  HDL ROM/1(data_out) -> data_out/1
  read_en/1 -> InputReg/2
  InputReg/1 -> HDL ROM/1(rom_address)
  address/1 -> InputReg/1

== system tx2/Subsystem10/OFDM_process1/OFDM_process1_bf1 ==
  data : Inport
  BF_ctrl : Inport  Port=2
  OFDM_BF1 : Subsystem
  ctrl_gen : Subsystem
  OFDM_process : Outport
  OFDM_ctrl_process : Outport  Port=2
  wires:
  ctrl_gen/1(data_out) -> OFDM_process/1  "OFDM_bf1_process1"
  BF_ctrl/1 -> OFDM_BF1/2(OFDM_ctrl)
  ctrl_gen/2(ctrl_out) -> OFDM_ctrl_process/1  "OFDM_ctrl_bf1_process1"
  data/1 -> OFDM_BF1/1(data)
  OFDM_BF1/2(valid_out) -> ctrl_gen/2(valid_in)
  OFDM_BF1/1(data_out) -> ctrl_gen/1(data_in)

== system tx2/Subsystem10/OFDM_process1/OFDM_process1_bf2 ==
  data : Inport
  BF_ctrl : Inport  Port=2
  OFDM_BF1 : Subsystem
  ctrl_gen : Subsystem
  OFDM_process : Outport
  OFDM_ctrl_process : Outport  Port=2
  wires:
  OFDM_BF1/1(data_out) -> ctrl_gen/1(data_in)
  OFDM_BF1/2(valid_out) -> ctrl_gen/2(valid_in)
  data/1 -> OFDM_BF1/1(data)
  ctrl_gen/2(ctrl_out) -> OFDM_ctrl_process/1  "OFDM_ctrl_bf1_process1"
  BF_ctrl/1 -> OFDM_BF1/2(OFDM_ctrl)
  ctrl_gen/1(data_out) -> OFDM_process/1  "OFDM_bf1_process1"

== system tx2/Subsystem10/OFDM_process1/OFDM_process1_bf3 ==
  data : Inport
  BF_ctrl : Inport  Port=2
  OFDM_BF1 : Subsystem
  ctrl_gen : Subsystem
  OFDM_process : Outport
  OFDM_ctrl_process : Outport  Port=2
  wires:
  ctrl_gen/1(data_out) -> OFDM_process/1  "OFDM_bf1_process1"
  BF_ctrl/1 -> OFDM_BF1/2(OFDM_ctrl)
  ctrl_gen/2(ctrl_out) -> OFDM_ctrl_process/1  "OFDM_ctrl_bf1_process1"
  data/1 -> OFDM_BF1/1(data)
  OFDM_BF1/2(valid_out) -> ctrl_gen/2(valid_in)
  OFDM_BF1/1(data_out) -> ctrl_gen/1(data_in)

== system tx2/Subsystem10/OFDM_process1/OFDM_process1_bf4 ==
  data : Inport
  BF_ctrl : Inport  Port=2
  OFDM_BF1 : Subsystem
  ctrl_gen : Subsystem
  OFDM_process : Outport
  OFDM_ctrl_process : Outport  Port=2
  wires:
  OFDM_BF1/1(data_out) -> ctrl_gen/1(data_in)
  OFDM_BF1/2(valid_out) -> ctrl_gen/2(valid_in)
  data/1 -> OFDM_BF1/1(data)
  ctrl_gen/2(ctrl_out) -> OFDM_ctrl_process/1  "OFDM_ctrl_bf1_process1"
  BF_ctrl/1 -> OFDM_BF1/2(OFDM_ctrl)
  ctrl_gen/1(data_out) -> OFDM_process/1  "OFDM_bf1_process1"

== system tx2/Subsystem10/OFDM_process1/OFDM_process1_bf5 ==
  data : Inport
  BF_ctrl : Inport  Port=2
  OFDM_BF1 : Subsystem
  ctrl_gen : Subsystem
  OFDM_process : Outport
  OFDM_ctrl_process : Outport  Port=2
  wires:
  ctrl_gen/1(data_out) -> OFDM_process/1  "OFDM_bf1_process1"
  BF_ctrl/1 -> OFDM_BF1/2(OFDM_ctrl)
  ctrl_gen/2(ctrl_out) -> OFDM_ctrl_process/1  "OFDM_ctrl_bf1_process1"
  data/1 -> OFDM_BF1/1(data)
  OFDM_BF1/2(valid_out) -> ctrl_gen/2(valid_in)
  OFDM_BF1/1(data_out) -> ctrl_gen/1(data_in)

== system tx2/Subsystem10/OFDM_process1/OFDM_process1_bf6 ==
  data : Inport
  BF_ctrl : Inport  Port=2
  OFDM_BF1 : Subsystem
  ctrl_gen : Subsystem
  OFDM_process : Outport
  OFDM_ctrl_process : Outport  Port=2
  wires:
  OFDM_BF1/1(data_out) -> ctrl_gen/1(data_in)
  OFDM_BF1/2(valid_out) -> ctrl_gen/2(valid_in)
  data/1 -> OFDM_BF1/1(data)
  ctrl_gen/2(ctrl_out) -> OFDM_ctrl_process/1  "OFDM_ctrl_bf1_process1"
  BF_ctrl/1 -> OFDM_BF1/2(OFDM_ctrl)
  ctrl_gen/1(data_out) -> OFDM_process/1  "OFDM_bf1_process1"

== system tx2/Subsystem10/OFDM_process1/OFDM_process1_bf7 ==
  data : Inport
  BF_ctrl : Inport  Port=2
  OFDM_BF1 : Subsystem
  ctrl_gen : Subsystem
  OFDM_process : Outport
  OFDM_ctrl_process : Outport  Port=2
  wires:
  ctrl_gen/1(data_out) -> OFDM_process/1  "OFDM_bf1_process1"
  BF_ctrl/1 -> OFDM_BF1/2(OFDM_ctrl)
  ctrl_gen/2(ctrl_out) -> OFDM_ctrl_process/1  "OFDM_ctrl_bf1_process1"
  data/1 -> OFDM_BF1/1(data)
  OFDM_BF1/2(valid_out) -> ctrl_gen/2(valid_in)
  OFDM_BF1/1(data_out) -> ctrl_gen/1(data_in)

== system tx2/Subsystem10/OFDM_process1/OFDM_process1_bf8 ==
  data : Inport
  BF_ctrl : Inport  Port=2
  OFDM_BF1 : Subsystem
  ctrl_gen : Subsystem
  OFDM_process : Outport
  OFDM_ctrl_process : Outport  Port=2
  wires:
  OFDM_BF1/1(data_out) -> ctrl_gen/1(data_in)
  OFDM_BF1/2(valid_out) -> ctrl_gen/2(valid_in)
  data/1 -> OFDM_BF1/1(data)
  ctrl_gen/2(ctrl_out) -> OFDM_ctrl_process/1  "OFDM_ctrl_bf1_process1"
  BF_ctrl/1 -> OFDM_BF1/2(OFDM_ctrl)
  ctrl_gen/1(data_out) -> OFDM_process/1  "OFDM_bf1_process1"

== system tx2/Subsystem10/bit_level/Subsystem ==
  end_in : Inport  OutDataTypeStr=boolean
  Data Type Conversion : DataTypeConversion  OutDataTypeStr=boolean  SaturateOnIntegerOverflow=off  RndMeth=Floor
  HDL Counter : hdlsllib/Sources/HDL Counter  CountType=Count limited  CountInit=1  CountStep=1  CountMax=192  CountFromType=Initial value  CountFrom=1  CountResetPort=on  CountLoadPort=off  CountEnbPort=off  CountDirPort=off  CountHitOutputPort=on  CountDataType=Unsigned  CountWordLen=8  CountFracLen=0  CountSampTime=1
  HDL Counter1 : hdlsllib/Sources/HDL Counter  CountType=Count limited  CountInit=0  CountStep=1  CountMax=1  CountFromType=Initial value  CountFrom=0  CountResetPort=on  CountLoadPort=off  CountEnbPort=on  CountDirPort=off  CountHitOutputPort=off  CountDataType=Unsigned  CountWordLen=1  CountFracLen=0  CountSampTime=1
  Logical Operator : Logic  AllPortsSameDT=off  OutDataTypeStr=boolean
  end_out : Outport  OutDataTypeStr=boolean
  wires:
  Logical Operator/1 -> end_out/1
  HDL Counter/2 -> HDL Counter1/1, Logical Operator/1
  Data Type Conversion/1 -> Logical Operator/2
  end_in/1 -> HDL Counter1/2, HDL Counter/1
  HDL Counter1/1 -> Data Type Conversion/1

== system tx2/Subsystem10/bit_level/ctrl_gen ==
  data_in : Inport
  select_valid : Inport  Port=2  OutDataTypeStr=boolean
  Constant : Constant  Value=0  OutDataTypeStr=boolean
  Switch : Switch  Criteria=u2 ~= 0  SaturateOnIntegerOverflow=off  InputSameDT=off
  ctrl_gen : Subsystem
  data_out : Outport
  ctrl_out : Outport  Port=2
  wires:
  data_in/1 -> Switch/1
  ctrl_gen/2(ctrl_out) -> ctrl_out/1
  ctrl_gen/1(data_out) -> data_out/1
  select_valid/1 -> Switch/2, ctrl_gen/2(valid_in)
  Constant/1 -> Switch/3
  Switch/1 -> ctrl_gen/1(data_in)

== system tx2/Subsystem10/bit_level/valid_recover ==
  data_in : Inport
  start_in : Inport  Port=2
  end_in : Inport  Port=3
  Constant : Constant  OutDataTypeStr=boolean
  Constant1 : Constant  Value=0  OutDataTypeStr=boolean
  Constant2 : Constant  OutDataTypeStr=boolean
  Constant3 : Constant  Value=0  OutDataTypeStr=boolean
  Constant4 : Constant  OutDataTypeStr=boolean
  Constant5 : Constant  Value=0  OutDataTypeStr=boolean
  Delay{,1..4} (5 alike) : Delay  DelayLength=1  InitialCondition=0
  Logical Operator1 : Logic  Operator=OR  AllPortsSameDT=off  OutDataTypeStr=boolean
  Logical Operator2 : Logic  AllPortsSameDT=off  OutDataTypeStr=boolean
  Switch : Switch  Criteria=u2 ~= 0  SaturateOnIntegerOverflow=off  InputSameDT=off
  Switch1 : Switch  Criteria=u2 ~= 0  SaturateOnIntegerOverflow=off  InputSameDT=off
  Switch2 : Switch  Criteria=u2 ~= 0  SaturateOnIntegerOverflow=off  InputSameDT=off
  data_out : Outport  VectorParamsAs1DForOutWhenUnconnected=off
  start_out : Outport  Port=2  VectorParamsAs1DForOutWhenUnconnected=off
  end_out : Outport  Port=3  VectorParamsAs1DForOutWhenUnconnected=off
  valid_out : Outport  Port=4  VectorParamsAs1DForOutWhenUnconnected=off
  wires:
  Constant/1 -> Switch/1
  Constant2/1 -> Switch1/3
  Switch/1 -> Logical Operator1/2
  Switch1/1 -> Logical Operator2/2
  Delay/1 -> start_out/1, Switch/2
  Delay2/1 -> Switch1/2
  Logical Operator1/1 -> Logical Operator2/1
  Switch2/1 -> Logical Operator1/1
  Delay3/1 -> Switch2/2
  Constant5/1 -> Switch2/3
  Constant4/1 -> Switch2/1
  start_in/1 -> Delay/1
  Constant3/1 -> Switch1/1
  Logical Operator2/1 -> valid_out/1, Delay3/1
  Constant1/1 -> Switch/3
  end_in/1 -> Delay1/1
  Delay1/1 -> end_out/1, Delay2/1
  data_in/1 -> Delay4/1
  Delay4/1 -> data_out/1

== system tx2/Subsystem11/BF/rom_bf1 ==
  address : Inport
  read_en : Inport  Port=2
  HDL ROM : Subsystem
  InputReg : Delay  DelayLength=1  ShowEnablePort=on
      settings: InputPortMap=u0,e6
  data_out : Outport
  wires:
  address/1 -> InputReg/1
  InputReg/1 -> HDL ROM/1(rom_address)
  read_en/1 -> InputReg/2
  HDL ROM/1(data_out) -> data_out/1

== system tx2/Subsystem11/BF/rom_bf2 ==
  address : Inport
  read_en : Inport  Port=2
  HDL ROM : Subsystem
  InputReg : Delay  DelayLength=1  ShowEnablePort=on
      settings: InputPortMap=u0,e6
  data_out : Outport
  wires:
  HDL ROM/1(data_out) -> data_out/1
  read_en/1 -> InputReg/2
  InputReg/1 -> HDL ROM/1(rom_address)
  address/1 -> InputReg/1

== system tx2/Subsystem11/BF/rom_bf3 ==
  address : Inport
  read_en : Inport  Port=2
  HDL ROM : Subsystem
  InputReg : Delay  DelayLength=1  ShowEnablePort=on
      settings: InputPortMap=u0,e6
  data_out : Outport
  wires:
  address/1 -> InputReg/1
  InputReg/1 -> HDL ROM/1(rom_address)
  read_en/1 -> InputReg/2
  HDL ROM/1(data_out) -> data_out/1

== system tx2/Subsystem11/BF/rom_bf4 ==
  address : Inport
  read_en : Inport  Port=2
  HDL ROM : Subsystem
  InputReg : Delay  DelayLength=1  ShowEnablePort=on
      settings: InputPortMap=u0,e6
  data_out : Outport
  wires:
  HDL ROM/1(data_out) -> data_out/1
  read_en/1 -> InputReg/2
  InputReg/1 -> HDL ROM/1(rom_address)
  address/1 -> InputReg/1

== system tx2/Subsystem11/BF/rom_bf5 ==
  address : Inport
  read_en : Inport  Port=2
  HDL ROM : Subsystem
  InputReg : Delay  DelayLength=1  ShowEnablePort=on
      settings: InputPortMap=u0,e6
  data_out : Outport
  wires:
  address/1 -> InputReg/1
  InputReg/1 -> HDL ROM/1(rom_address)
  read_en/1 -> InputReg/2
  HDL ROM/1(data_out) -> data_out/1

== system tx2/Subsystem11/BF/rom_bf6 ==
  address : Inport
  read_en : Inport  Port=2
  HDL ROM : Subsystem
  InputReg : Delay  DelayLength=1  ShowEnablePort=on
      settings: InputPortMap=u0,e6
  data_out : Outport
  wires:
  HDL ROM/1(data_out) -> data_out/1
  read_en/1 -> InputReg/2
  InputReg/1 -> HDL ROM/1(rom_address)
  address/1 -> InputReg/1

== system tx2/Subsystem11/BF/rom_bf7 ==
  address : Inport
  read_en : Inport  Port=2
  HDL ROM : Subsystem
  InputReg : Delay  DelayLength=1  ShowEnablePort=on
      settings: InputPortMap=u0,e6
  data_out : Outport
  wires:
  address/1 -> InputReg/1
  InputReg/1 -> HDL ROM/1(rom_address)
  read_en/1 -> InputReg/2
  HDL ROM/1(data_out) -> data_out/1

== system tx2/Subsystem11/BF/rom_bf8 ==
  address : Inport
  read_en : Inport  Port=2
  HDL ROM : Subsystem
  InputReg : Delay  DelayLength=1  ShowEnablePort=on
      settings: InputPortMap=u0,e6
  data_out : Outport
  wires:
  HDL ROM/1(data_out) -> data_out/1
  read_en/1 -> InputReg/2
  InputReg/1 -> HDL ROM/1(rom_address)
  address/1 -> InputReg/1

== system tx2/Subsystem11/OFDM_process1/OFDM_process1_bf1 ==
  data : Inport
  BF_ctrl : Inport  Port=2
  OFDM_BF1 : Subsystem
  ctrl_gen : Subsystem
  OFDM_process : Outport
  OFDM_ctrl_process : Outport  Port=2
  wires:
  OFDM_BF1/1(data_out) -> ctrl_gen/1(data_in)
  OFDM_BF1/2(valid_out) -> ctrl_gen/2(valid_in)
  data/1 -> OFDM_BF1/1(data)
  ctrl_gen/2(ctrl_out) -> OFDM_ctrl_process/1  "OFDM_ctrl_bf1_process1"
  BF_ctrl/1 -> OFDM_BF1/2(OFDM_ctrl)
  ctrl_gen/1(data_out) -> OFDM_process/1  "OFDM_bf1_process1"

== system tx2/Subsystem11/OFDM_process1/OFDM_process1_bf2 ==
  data : Inport
  BF_ctrl : Inport  Port=2
  OFDM_BF1 : Subsystem
  ctrl_gen : Subsystem
  OFDM_process : Outport
  OFDM_ctrl_process : Outport  Port=2
  wires:
  ctrl_gen/1(data_out) -> OFDM_process/1  "OFDM_bf1_process1"
  BF_ctrl/1 -> OFDM_BF1/2(OFDM_ctrl)
  ctrl_gen/2(ctrl_out) -> OFDM_ctrl_process/1  "OFDM_ctrl_bf1_process1"
  data/1 -> OFDM_BF1/1(data)
  OFDM_BF1/2(valid_out) -> ctrl_gen/2(valid_in)
  OFDM_BF1/1(data_out) -> ctrl_gen/1(data_in)

== system tx2/Subsystem11/OFDM_process1/OFDM_process1_bf3 ==
  data : Inport
  BF_ctrl : Inport  Port=2
  OFDM_BF1 : Subsystem
  ctrl_gen : Subsystem
  OFDM_process : Outport
  OFDM_ctrl_process : Outport  Port=2
  wires:
  OFDM_BF1/1(data_out) -> ctrl_gen/1(data_in)
  OFDM_BF1/2(valid_out) -> ctrl_gen/2(valid_in)
  data/1 -> OFDM_BF1/1(data)
  ctrl_gen/2(ctrl_out) -> OFDM_ctrl_process/1  "OFDM_ctrl_bf1_process1"
  BF_ctrl/1 -> OFDM_BF1/2(OFDM_ctrl)
  ctrl_gen/1(data_out) -> OFDM_process/1  "OFDM_bf1_process1"

== system tx2/Subsystem11/OFDM_process1/OFDM_process1_bf4 ==
  data : Inport
  BF_ctrl : Inport  Port=2
  OFDM_BF1 : Subsystem
  ctrl_gen : Subsystem
  OFDM_process : Outport
  OFDM_ctrl_process : Outport  Port=2
  wires:
  ctrl_gen/1(data_out) -> OFDM_process/1  "OFDM_bf1_process1"
  BF_ctrl/1 -> OFDM_BF1/2(OFDM_ctrl)
  ctrl_gen/2(ctrl_out) -> OFDM_ctrl_process/1  "OFDM_ctrl_bf1_process1"
  data/1 -> OFDM_BF1/1(data)
  OFDM_BF1/2(valid_out) -> ctrl_gen/2(valid_in)
  OFDM_BF1/1(data_out) -> ctrl_gen/1(data_in)

== system tx2/Subsystem11/OFDM_process1/OFDM_process1_bf5 ==
  data : Inport
  BF_ctrl : Inport  Port=2
  OFDM_BF1 : Subsystem
  ctrl_gen : Subsystem
  OFDM_process : Outport
  OFDM_ctrl_process : Outport  Port=2
  wires:
  OFDM_BF1/1(data_out) -> ctrl_gen/1(data_in)
  OFDM_BF1/2(valid_out) -> ctrl_gen/2(valid_in)
  data/1 -> OFDM_BF1/1(data)
  ctrl_gen/2(ctrl_out) -> OFDM_ctrl_process/1  "OFDM_ctrl_bf1_process1"
  BF_ctrl/1 -> OFDM_BF1/2(OFDM_ctrl)
  ctrl_gen/1(data_out) -> OFDM_process/1  "OFDM_bf1_process1"

== system tx2/Subsystem11/OFDM_process1/OFDM_process1_bf6 ==
  data : Inport
  BF_ctrl : Inport  Port=2
  OFDM_BF1 : Subsystem
  ctrl_gen : Subsystem
  OFDM_process : Outport
  OFDM_ctrl_process : Outport  Port=2
  wires:
  ctrl_gen/1(data_out) -> OFDM_process/1  "OFDM_bf1_process1"
  BF_ctrl/1 -> OFDM_BF1/2(OFDM_ctrl)
  ctrl_gen/2(ctrl_out) -> OFDM_ctrl_process/1  "OFDM_ctrl_bf1_process1"
  data/1 -> OFDM_BF1/1(data)
  OFDM_BF1/2(valid_out) -> ctrl_gen/2(valid_in)
  OFDM_BF1/1(data_out) -> ctrl_gen/1(data_in)

== system tx2/Subsystem11/OFDM_process1/OFDM_process1_bf7 ==
  data : Inport
  BF_ctrl : Inport  Port=2
  OFDM_BF1 : Subsystem
  ctrl_gen : Subsystem
  OFDM_process : Outport
  OFDM_ctrl_process : Outport  Port=2
  wires:
  OFDM_BF1/1(data_out) -> ctrl_gen/1(data_in)
  OFDM_BF1/2(valid_out) -> ctrl_gen/2(valid_in)
  data/1 -> OFDM_BF1/1(data)
  ctrl_gen/2(ctrl_out) -> OFDM_ctrl_process/1  "OFDM_ctrl_bf1_process1"
  BF_ctrl/1 -> OFDM_BF1/2(OFDM_ctrl)
  ctrl_gen/1(data_out) -> OFDM_process/1  "OFDM_bf1_process1"

== system tx2/Subsystem11/OFDM_process1/OFDM_process1_bf8 ==
  data : Inport
  BF_ctrl : Inport  Port=2
  OFDM_BF1 : Subsystem
  ctrl_gen : Subsystem
  OFDM_process : Outport
  OFDM_ctrl_process : Outport  Port=2
  wires:
  ctrl_gen/1(data_out) -> OFDM_process/1  "OFDM_bf1_process1"
  BF_ctrl/1 -> OFDM_BF1/2(OFDM_ctrl)
  ctrl_gen/2(ctrl_out) -> OFDM_ctrl_process/1  "OFDM_ctrl_bf1_process1"
  data/1 -> OFDM_BF1/1(data)
  OFDM_BF1/2(valid_out) -> ctrl_gen/2(valid_in)
  OFDM_BF1/1(data_out) -> ctrl_gen/1(data_in)

== system tx2/Subsystem11/bit_level/Subsystem ==
  end_in : Inport  OutDataTypeStr=boolean
  Data Type Conversion : DataTypeConversion  OutDataTypeStr=boolean  SaturateOnIntegerOverflow=off  RndMeth=Floor
  HDL Counter : hdlsllib/Sources/HDL Counter  CountType=Count limited  CountInit=1  CountStep=1  CountMax=192  CountFromType=Initial value  CountFrom=1  CountResetPort=on  CountLoadPort=off  CountEnbPort=off  CountDirPort=off  CountHitOutputPort=on  CountDataType=Unsigned  CountWordLen=8  CountFracLen=0  CountSampTime=1
  HDL Counter1 : hdlsllib/Sources/HDL Counter  CountType=Count limited  CountInit=0  CountStep=1  CountMax=1  CountFromType=Initial value  CountFrom=0  CountResetPort=on  CountLoadPort=off  CountEnbPort=on  CountDirPort=off  CountHitOutputPort=off  CountDataType=Unsigned  CountWordLen=1  CountFracLen=0  CountSampTime=1
  Logical Operator : Logic  AllPortsSameDT=off  OutDataTypeStr=boolean
  end_out : Outport  OutDataTypeStr=boolean
  wires:
  HDL Counter1/1 -> Data Type Conversion/1
  end_in/1 -> HDL Counter/1, HDL Counter1/2
  Data Type Conversion/1 -> Logical Operator/2
  HDL Counter/2 -> Logical Operator/1, HDL Counter1/1
  Logical Operator/1 -> end_out/1

== system tx2/Subsystem11/bit_level/ctrl_gen ==
  data_in : Inport
  select_valid : Inport  Port=2  OutDataTypeStr=boolean
  Constant : Constant  Value=0  OutDataTypeStr=boolean
  Switch : Switch  Criteria=u2 ~= 0  SaturateOnIntegerOverflow=off  InputSameDT=off
  ctrl_gen : Subsystem
  data_out : Outport
  ctrl_out : Outport  Port=2
  wires:
  Switch/1 -> ctrl_gen/1(data_in)
  Constant/1 -> Switch/3
  select_valid/1 -> ctrl_gen/2(valid_in), Switch/2
  ctrl_gen/1(data_out) -> data_out/1
  ctrl_gen/2(ctrl_out) -> ctrl_out/1
  data_in/1 -> Switch/1
